simulink subsystem "exhaust_lut_controller"  (R2024b)
settings: Solver=VariableStepAuto  StartTime=0.0  StopTime=10.0  RelTol=1e-3
undefined symbols (not defined in the file): baro_lut, const_brake, controller_rate
settings Model: Creator=yevge  LastModifiedBy=Yevgeniy Gorbachev

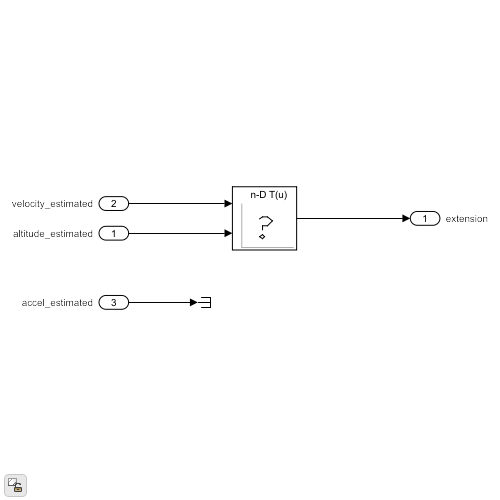
[thumbnail: Simulink's stored preview of the top-level diagram]
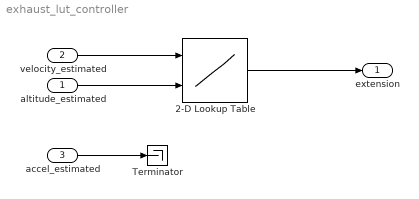
== system exhaust_lut_controller ==
  altitude_estimated : Inport  Unit=m  PortDimensions=1
  velocity_estimated : Inport  Port=2  Unit=m/s  PortDimensions=1
  accel_estimated : Inport  Port=3  Unit=m/s^2  PortDimensions=1
  2-D Lookup Table : Lookup_n-D  DataSpecification=Lookup table object  LookupTableObject=baro_lut  BreakpointsForDimension1=baro_lut.vel  BreakpointsForDimension2=baro_lut.alt  Table=baro_lut{:, :}  InternalRulePriority=Speed  RndMeth=Simplest
      settings: InputPortMap=u0,u1
  Terminator : Terminator
  extension : Outport  OutMin=0  OutMax=1  Unit=1  PortDimensions=1  SampleTime=1/controller_rate  InitialOutput=const_brake
  wires:
  accel_estimated/1 -> Terminator/1
  velocity_estimated/1 -> 2-D Lookup Table/1
  altitude_estimated/1 -> 2-D Lookup Table/2
  2-D Lookup Table/1 -> extension/1
